simulink model "TOAD_StateEstimator"  (R2025b)
settings: Solver=VariableStepAuto  StartTime=0.0  StopTime=10.0  RelTol=1e-3
undefined symbols (not defined in the file): constantsTOAD, dt_SIM
settings Model: DataDictionary=Model_Vars.sldd  Creator=pplat  LastModifiedBy=pplat

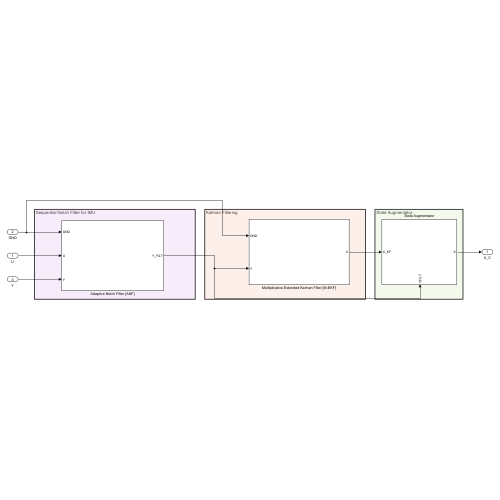
[thumbnail: Simulink's stored preview of the top-level diagram]
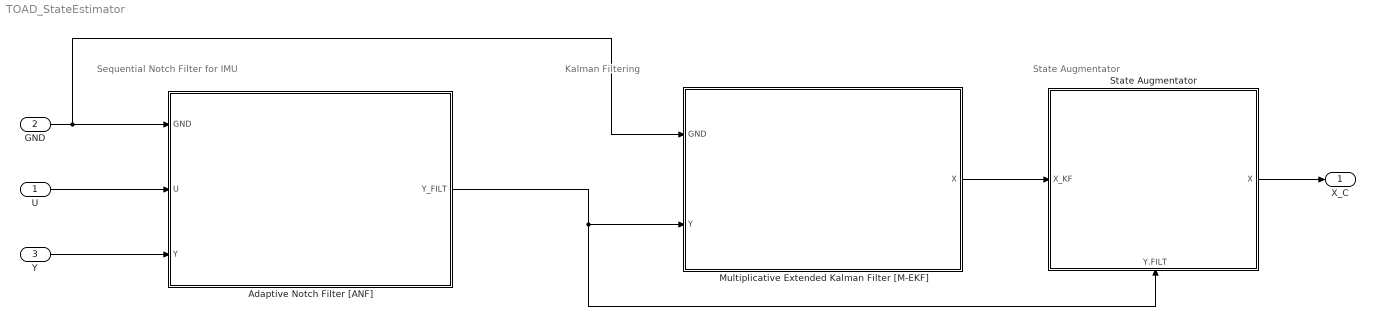
== system TOAD_StateEstimator ==
  note: Kalman Filtering
  note: State Augmentator
  note: Sequential Notch Filter for IMU
  U : Inport
  GND : Inport  Port=2
  Y : Inport  Port=3
  Adaptive Notch Filter [ANF] : Subsystem
  Multiplicative Extended Kalman Filter [M-EKF] : Subsystem
  State Augmentator : Subsystem
      settings: PortSchema="{\"entries\":[{\"content\":{\"sides\":[{\"content\":{\"connectorIds\":[\"In1\"]},\"type\":\"ConnectorPlacement.EquallySpacedRectSide\",\"uuid\":\"bb6458aa-622a-4d42-b468-f616d6e302fe\"},{\"content\":{\"connectorIds\":[\"Out1\"],\"side\":\"RIGHT\"},\"type\":\"ConnectorPlacement.EquallySpacedRectSide\",\"uuid\":\"af8bade2-eb0a-4714-9db5-d33244eb3558\"},{\"content\":{\"side\":\"TOP\"},\"type\":\"ConnectorPlacement.EquallySpacedRectSide\",\"uuid\":\"05a7f106-e447-475e-b3b5-727cb0579a7b\"},{\"content\":{\"connectorIds\":[\"In2\"],\"side\":\"BOTTOM\"},\"type\":\"ConnectorPlacement.EquallySpacedRectSide\",\"uuid\":\"a6d44455-a42d-44f7-b37b-0d3db398c8f2\"}]},\"type\":\"ConnectorPlacement.EquallySpacedConnector\",\"uuid\":\"c6f62579-6b17-43b5-92f1-6190f0d9fd8b\"}],\"packageUris\":[\"http://schema.mathworks.com/mf0/Connector/R2020b\"],\"version\":\"1.0\"}"
  X_C : Outport
  wires:
  U/1 -> Adaptive Notch Filter [ANF]/2(U)
  Adaptive Notch Filter [ANF]/1(Y_FILT) -> State Augmentator/2(Y.FILT), Multiplicative Extended Kalman Filter [M-EKF]/2(Y)
  GND/1 -> Adaptive Notch Filter [ANF]/1(GND), Multiplicative Extended Kalman Filter [M-EKF]/1(GND)
  State Augmentator/1(X) -> X_C/1
  Multiplicative Extended Kalman Filter [M-EKF]/1(X) -> State Augmentator/1(X_KF)
  Y/1 -> Adaptive Notch Filter [ANF]/3(Y)

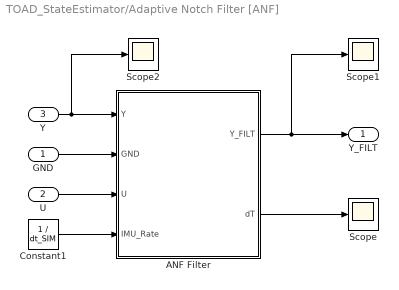
== system TOAD_StateEstimator/Adaptive Notch Filter [ANF] ==
  GND : Inport
  U : Inport  Port=2
  Y : Inport  Port=3
  ANF Filter : MATLAB Function  TreatAsAtomicUnit=on
  Constant1 : Constant  Value=1 / dt_SIM
  Scope : Scope
      settings: ActiveDisplayYMinimum=0.00097880622837365075  ActiveDisplayYMaximum=0.0020384948096911198  DataLoggingVariableName=ScopeData12
  Scope1 : Scope
      settings: ActiveDisplayYMinimum=9.4335953871319269  ActiveDisplayYMaximum=11.786797462805113  DataLoggingVariableName=ScopeData15
  Scope2 : Scope
      settings: ActiveDisplayYMinimum=-0.822722965610661  ActiveDisplayYMaximum=0.985135629551039  DataLoggingVariableName=ScopeData16
  Y_FILT : Outport
  wires:
  ANF Filter/1(Y_FILT) -> Scope1/1, Y_FILT/1
  GND/1 -> ANF Filter/2(GND)
  U/1 -> ANF Filter/3(U)
  Y/1 -> Scope2/1, ANF Filter/1(Y)
  Constant1/1 -> ANF Filter/4(IMU_Rate)
  ANF Filter/2(dT) -> Scope/1

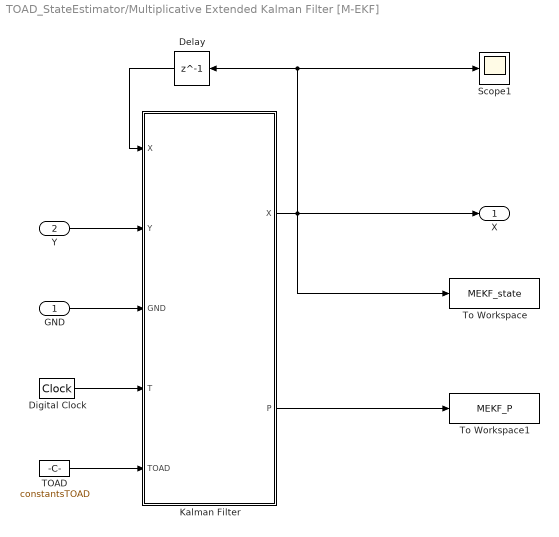
== system TOAD_StateEstimator/Multiplicative Extended Kalman Filter [M-EKF] ==
  GND : Inport
  Y : Inport  Port=2
  Delay : Delay  DelayLength=1  InitialCondition=[1; zeros(18,1)]
  Digital Clock : DigitalClock  SampleTime=dt_SIM
  Kalman Filter : MATLAB Function  TreatAsAtomicUnit=on
  Scope1 : Scope
      settings: ActiveDisplayYMinimum=-11.196961871902474  ActiveDisplayYMaximum=4.52812403188117  DataLoggingVariableName=ScopeData11
  TOAD : Constant  Value=constantsTOAD  OutDataTypeStr=Bus: slBus1
  To Workspace : ToWorkspace  VariableName=MEKF_state  SaveFormat=Timeseries  SampleTime=-1
  To Workspace1 : ToWorkspace  VariableName=MEKF_P  SaveFormat=Timeseries  SampleTime=-1
  X : Outport
  wires:
  Digital Clock/1 -> Kalman Filter/4(T)
  Kalman Filter/1(X) -> To Workspace/1, Scope1/1, Delay/1, X/1
  Y/1 -> Kalman Filter/2(Y)
  Delay/1 -> Kalman Filter/1("X ")
  TOAD/1 -> Kalman Filter/5(TOAD)
  GND/1 -> Kalman Filter/3(GND)
  Kalman Filter/2(P) -> To Workspace1/1

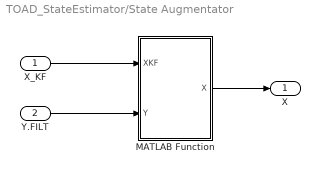
== system TOAD_StateEstimator/State Augmentator ==
  X_KF : Inport
  Y.FILT : Inport  Port=2
  MATLAB Function : MATLAB Function  TreatAsAtomicUnit=on
  X : Outport
  wires:
  X_KF/1 -> MATLAB Function/1(XKF)
  MATLAB Function/1(X) -> X/1
  Y.FILT/1 -> MATLAB Function/2(Y)

== matlab function TOAD_StateEstimator/Multiplicative Extended Kalman Filter [M-EKF]/Kalman Filter ==
  data: X input; Y input; GND input; X output; T input; TOAD input; P output
function [X, P] = MEKF(X, Y, GND, T, TOAD)

    % Measure simulation timestep
    persistent dt lastT lastP
    if isempty(dt)
        dt = 0;
        lastT = 0;
        lastP = eye(18);
    end
    dt = T - lastT;
    lastT = T;
    
    if GND
        [X, lastP] = GroundEstimator(X, TOAD, Y, dt);
    else
        [X, lastP(1:9, 1:9)] = FlightEstimator(X, TOAD, Y, dt, lastP(1:9, 1:9));
    end
    P = diag(lastP);
end
    %X = EstimateStateFCN(X, ASTRAv2, Y, dt, GND);

== matlab function TOAD_StateEstimator/State Augmentator/MATLAB Function ==
  data: XKF input; X output; Y input
function X = StateAUG(XKF, Y)

% Change Filter State to Controls State
X = [XKF(1:4); XKF(5:7); XKF(8:10); Y(4:6) - XKF(11:13); XKF(11:13)];

== matlab function TOAD_StateEstimator/Adaptive Notch Filter [ANF]/ANF Filter ==
  data: Y input; Y_FILT output; GND input; U input; IMU_Rate input; dT output
function [Y_FILT, dT] = ANF_Filter(Y, GND, U, IMU_Rate)

% Extract IMU
IMU = Y(1:9);
dT = 1 / IMU_Rate;

% Thrust PCT
THRUST = U(3) / (1.697 * 9.80145) * 100;

% ANF Filter
ANF_IMU = DigitalNF(IMU, GND, THRUST, dT);

% Combine (FILTER CURRENTLY OFF)
Y_FILT = [ANF_IMU; Y(10:15)];
